simulink model "MRAC_P1_DZ"  (R2019b)
settings: Solver=VariableStepAuto  StartTime=0.0  StopTime=2000  RelTol=1e-3
undefined symbols (not defined in the file): sigbuilder_block
libraries: slctrlblks x3, simulink x2
settings Model: Creator=Henry  LastModifiedBy=Kevin
settings SFSimCC: CustomCodeUndefinedFunction=UseInterfaceOnly

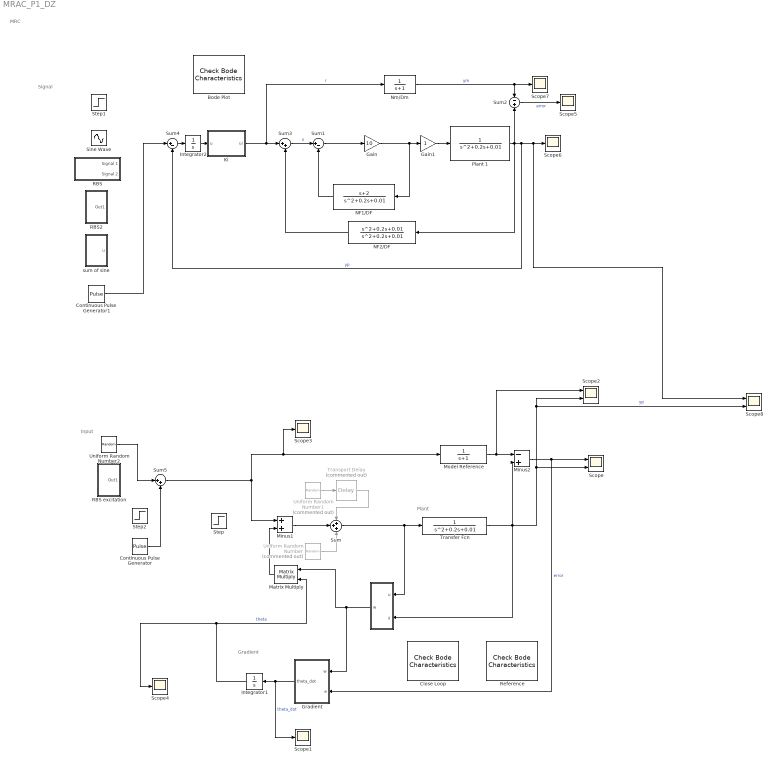
== system MRAC_P1_DZ ==
  note: Plant
  note: Gradient
  note: Signal
  note: MRC
  note: Input
  " " : Subsystem
  Bode Plot : slctrlblks/Model Verification/Check Bode  Characteristics  InstantiateOnLoad=on  SaveOperatingPoints=off  LinearizationIOs={'/Gain1', 1, 'in', 'off', '';'/Plant 1', 1, 'out', 'on', ''}  LinearizeAt=SnapshotTimes  SnapshotTimes=[0]  TriggerType=rising  SampleTime=auto  RateConversionMethod=zoh  PreWarpFreq=10  UseExactDelayModel=off  UseFullBlockNameLabels=off  UseBusSignalLabels=off  enabled=on  stopWhenAssertionFail=off  export=off  ViewDlgPos=[1981 -205.666666666667 1445.33333333333 714]  OpenViewOnLoad=off  LaunchViewOnOpen=off  FrequencyUnits=rad/s  MagnitudeUnits=dB  PhaseUnits=deg  TimeUnits=seconds  EnableUpperBound=off  UpperBoundFrequencies=[]  UpperBoundMagnitudes=[]  EnableLowerBound=off  LowerBoundFrequencies=[]  LowerBoundMagnitudes=[]
      settings: SourceProductName=Simulink Control Design
  Close Loop : slctrlblks/Model Verification/Check Bode  Characteristics  InstantiateOnLoad=on  SaveOperatingPoints=off  LinearizationIOs={'/Transfer Fcn', 1, 'out', 'off', '';'/Minus1', 1, 'in', 'off', ''}  LinearizeAt=SnapshotTimes  SnapshotTimes=[0]  TriggerType=rising  SampleTime=auto  RateConversionMethod=zoh  PreWarpFreq=10  UseExactDelayModel=off  UseFullBlockNameLabels=off  UseBusSignalLabels=off  enabled=on  stopWhenAssertionFail=off  export=off  ViewDlgPos=[100 200 510 390]  OpenViewOnLoad=off  LaunchViewOnOpen=on  FrequencyUnits=rad/s  MagnitudeUnits=dB  PhaseUnits=deg  TimeUnits=seconds  EnableUpperBound=off  UpperBoundFrequencies=[]  UpperBoundMagnitudes=[]  EnableLowerBound=off  LowerBoundFrequencies=[]  LowerBoundMagnitudes=[]
      settings: SourceProductName=Simulink Control Design
  Continuous Pulse Generator : DiscretePulseGenerator  PulseType=Time based  Period=100  PulseWidth=50
  Continuous Pulse Generator1 : DiscretePulseGenerator  PulseType=Time based  Period=100  PulseWidth=50
  Gain : Gain  Gain=10
  Gain1 : Gain
  Gradient : MATLAB Function  TreatAsAtomicUnit=on
  Integrator1 : Integrator
  Integrator2 : Integrator
  Ki : MATLAB Function  TreatAsAtomicUnit=on
  Matrix Multiply : Product  Multiplication=Matrix(*)
  Minus1 : Sum
  Minus2 : Sum  Inputs=-+
  Model Reference : TransferFcn  Denominator=[1 1]
  NF1/DF : TransferFcn  Numerator=[1 2]  Denominator=[1 0.2 0.01]
  NF2/DF : TransferFcn  Numerator=[1 0.2 0.01]  Denominator=[1 0.2 0.01]
  "Nm/Dm " : TransferFcn  Denominator=[1 1]
  Plant 1 : TransferFcn  Denominator=[1 ,0.2 ,0.01]
  "RBS " : Subsystem  Tag=STV Subsys  LoadFcn=sigbuilder_block('load');  StartFcn=sigbuilder_block('start');  StopFcn=sigbuilder_block('stop');  ClipboardFcn=sigbuilder_block('clipboard');  mask(Sigbuilder block){tuvar=[0:10]}
      mask help: Simulink:masks:SigbuilderBlock_MD
      mask init:
      | if ~strcmp(get_param(bdroot(gcbh),'SimulationStatus'),'stopped') tuvar = sigbuilder_block('maskInit'); end
      settings: CopyFcn=sigbuilder_block('copy');  DeleteFcn=sigbuilder_block('delete');  ModelCloseFcn=sigbuilder_block('modelClose');  PreSaveFcn=sigbuilder_block('preSave');  PauseFcn=sigbuilder_block('pause');  ContinueFcn=sigbuilder_block('continue');  NameChangeFcn=sigbuilder_block('namechange');  OpenFcn=sigbuilder_block('open',[215 62.5 550.5 362.5 ]);  CloseFcn=sigbuilder_block('close');
      mask Display: plot(0, 0, 100, 100,[2, 2, 32, 32, 2], [68, 8, 8, 68, 68],[32, 2], [38, 38], [32, 19, 2],[53, 60, 44], [32, 17, 17, 2],[16, 16, 31, 31]);txt = getActiveGroup(gcbh);text(2, 100, txt,'verticalAlignment', 'top');
  RBS excitation : Subsystem
  RBS2 : Subsystem
  Reference : slctrlblks/Model Verification/Check Bode  Characteristics  InstantiateOnLoad=on  SaveOperatingPoints=off  LinearizationIOs={'/Model Reference', 1, 'out', 'off', '';'/Step', 1, 'in', 'off', ''}  LinearizeAt=SnapshotTimes  SnapshotTimes=[0]  TriggerType=rising  SampleTime=auto  RateConversionMethod=zoh  PreWarpFreq=10  UseExactDelayModel=off  UseFullBlockNameLabels=off  UseBusSignalLabels=off  enabled=on  stopWhenAssertionFail=off  export=off  ViewDlgPos=[100 200 510 390]  OpenViewOnLoad=off  LaunchViewOnOpen=on  FrequencyUnits=rad/s  MagnitudeUnits=dB  PhaseUnits=deg  TimeUnits=seconds  EnableUpperBound=off  UpperBoundFrequencies=[]  UpperBoundMagnitudes=[]  EnableLowerBound=off  LowerBoundFrequencies=[]  LowerBoundMagnitudes=[]
      settings: SourceProductName=Simulink Control Design
  Scope : Scope  NumInputPorts=2
  Scope{1,3..7} (6 alike) : Scope
  Scope2 : Scope  NumInputPorts=2
  Scope8 : Scope  NumInputPorts=2
  Sine Wave : Sin  Frequency=0.1  SampleTime=0
  Step : Step  SampleTime=0
  Step1 : Step  SampleTime=0
  Step2 : Step  SampleTime=0
  Sum : Sum  Inputs=+++
  Sum1 : Sum  Inputs=|+-
  Sum2 : Sum  Inputs=-+
  Sum3 : Sum  Inputs=|++
  Sum4 : Sum  Inputs=|+-
  Sum5 : Sum  Inputs=|++
  Transfer Fcn : TransferFcn  Denominator=[1 ,0.2 ,0.01]
  Transport Delay : TransportDelay  Commented=on  DelayTime=150
  Uniform Random Number : UniformRandomNumber  Commented=on  SampleTime=0.05
  Uniform Random Number1 : UniformRandomNumber  Commented=on  Minimum=-5  Maximum=5  SampleTime=0.05
  Uniform Random Number2 : UniformRandomNumber  Minimum=-0.08  Maximum=0.08  SampleTime=1
  sum of sine : Subsystem
  wires:
  Model Reference/1 -> Scope2/1, Minus2/1
  Transfer Fcn/1 -> " "/2("y "), Scope8/2, Scope2/2, Scope/2, Minus2/2  "yp"
  Sum5/1 -> Minus1/1, Scope3/1, Model Reference/1
  Sum/1 -> " "/1("u "), Transfer Fcn/1
  Matrix Multiply/1 -> Minus1/2
  Gradient/1(theta_dot) -> Scope1/1, Integrator1/1  "theta_dot"
  " "/1(w) -> Gradient/1(w), Matrix Multiply/1
  Minus2/1 -> Scope/1, Gradient/2(e)  "error"
  Integrator1/1 -> Matrix Multiply/2, Scope4/1  "theta"
  Uniform Random Number/1 -> Sum/3
  Minus1/1 -> Sum/2
  Uniform Random Number1/1 -> Transport Delay/1
  Transport Delay/1 -> Sum/1
  NF1/DF/1 -> Sum1/2
  NF2/DF/1 -> Sum3/2
  Sum1/1 -> Gain/1
  Gain/1 -> Gain1/1, NF1/DF/1
  Sum4/1 -> Integrator2/1
  "Nm/Dm "/1 -> Scope7/1, Sum2/1  "ym"
  Gain1/1 -> Plant 1/1
  Ki/1(ui) -> "Nm/Dm "/1, Sum3/1  "r"
  Continuous Pulse Generator1/1 -> Sum4/1
  Sum3/1 -> Sum1/1  "u"
  Integrator2/1 -> Ki/1(u)
  Plant 1/1 -> Scope8/1, Scope6/1, Sum4/2, NF2/DF/1, Sum2/2  "yp"
  Sum2/1 -> Scope5/1  "error"
  Continuous Pulse Generator/1 -> Sum5/2
  Uniform Random Number2/1 -> Sum5/1

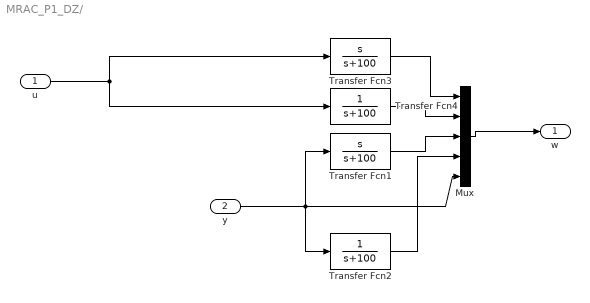
== system MRAC_P1_DZ/  ==
  "u " : Inport
  "y " : Inport  Port=2
  Mux : Mux  Inputs=5
  Transfer Fcn1 : TransferFcn  Numerator=[1 0]  Denominator=[1 100]
  Transfer Fcn2 : TransferFcn  Denominator=[1 100]
  Transfer Fcn3 : TransferFcn  Numerator=[1 0]  Denominator=[1 100]
  Transfer Fcn4 : TransferFcn  Denominator=[1 100]
  w : Outport
  wires:
  Transfer Fcn1/1 -> Mux/3
  "u "/1 -> Transfer Fcn3/1, Transfer Fcn4/1
  Mux/1 -> w/1
  "y "/1 -> Mux/5, Transfer Fcn2/1, Transfer Fcn1/1
  Transfer Fcn2/1 -> Mux/4
  Transfer Fcn3/1 -> Mux/1
  Transfer Fcn4/1 -> Mux/2

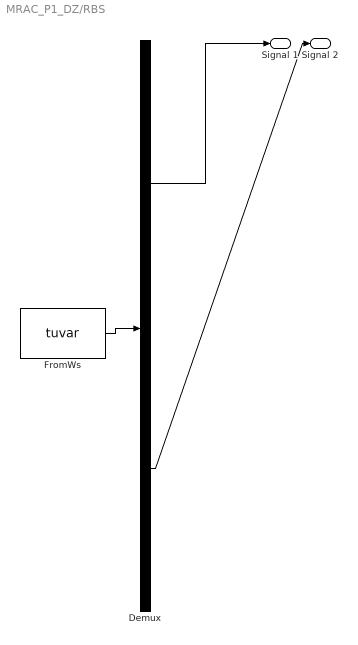
== system MRAC_P1_DZ/RBS  ==
  Demux : Demux  Tag=STV Demux  Outputs=2
  FromWs : FromWorkspace  Tag=STV FromWs  VariableName=tuvar  SampleTime=0
      SigBuilderData=|
      | common.afterFinalStr = 'Extrapolate'
      | common.sampleTime = 0
      | dataSet.timeRange = [0 10]
      | dataSet.name = 'Group 1'
      | sbobj.Groups.Name = 'Group 1'
      | sbobj.Groups.Signals(1).Name = 'Signal 1'
      | sbobj.Groups.Signals(1).XData = [0 4 4 6 6 10]
      | sbobj.Groups.Signals(1).YData = [0 0 1 1 0 0]
      | sbobj.Groups.Signals(2).Name = 'Signal 2'
      | sbobj.Groups.Signals(2).XData = [0 0.2 0.2 0.3 0.3 0.5 0.5 0.7 0.7 1 1 1.1 1.1 1.3 1.3 1.4 1.4 1.5 1.5 1.7 1.7 2.1 2.1 2.2 2.2 2.7 2.7 2.8 2.8 2.9 2.9 3 3 3.1 3.1 3.5 3.5 3.7 3.7 3.8 3.8 3.9 3.9 4.2 4.2 4.4 4.4 4.7 4.7 5 5 5.1 5.1 5.3 5.3 5.6 5.6 5.7 5.7 5.8 5.8 5.9 5.9 6 6 6.1 6.1 6.2 6.2 6.7 6.7 7 7 7.1 7.1 7.2 7.2 7.3 7.3 7.4 7.4 7.5 7.5 7.8 7.8 7.9 7.9 8.1 8.1 8.5 8.5 8.6 8.6 8.8 8.8 8.9 8.9 9 9 9.2 9.2 9.5 9.5 9.6 9.6 9.7 9.7 10]
      | sbobj.Groups.Signals(2).YData = [1 1 0 0 1 1 0 0 1 1 0 0 1 1 0 0 1 1 0 0 1 1 0 0 1 1 0 0 1 1 0 0 1 1 0 0 1 1 0 0 1 1 0 0 1 1 0 0 1 1 0 0 1 1 0 0 1 1 0 0 1 1 0 0 1 1 0 0 1 1 0 0 1 1 0 0 1 1 0 0 1 1 0 0 1 1 0 0 1 1 0 0 1 1 0 0 1 1 0 0 1 1 0 0 1 1 0 0]
  Signal 1 : Outport  Tag=STV Outport
  Signal 2 : Outport  Tag=STV Outport  Port=2
  wires:
  Demux/1 -> Signal 1/1
  FromWs/1 -> Demux/1
  Demux/2 -> Signal 2/1

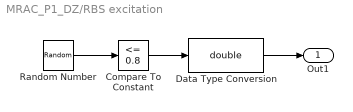
== system MRAC_P1_DZ/RBS excitation ==
  Compare To Constant : simulink/Logic and Bit Operations/Compare To Constant  relop=<=  const=0.8  OutDataTypeStr=boolean
  Data Type Conversion : DataTypeConversion  OutDataTypeStr=double
  Random Number : RandomNumber  Mean=1  SampleTime=10
  Out1 : Outport
  wires:
  Random Number/1 -> Compare To Constant/1
  Compare To Constant/1 -> Data Type Conversion/1
  Data Type Conversion/1 -> Out1/1

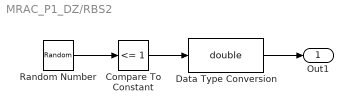
== system MRAC_P1_DZ/RBS2 ==
  Compare To Constant : simulink/Logic and Bit Operations/Compare To Constant  relop=<=  const=1  OutDataTypeStr=boolean
  Data Type Conversion : DataTypeConversion  OutDataTypeStr=double
  Random Number : RandomNumber  Mean=1  SampleTime=10
  Out1 : Outport
  wires:
  Random Number/1 -> Compare To Constant/1
  Compare To Constant/1 -> Data Type Conversion/1
  Data Type Conversion/1 -> Out1/1

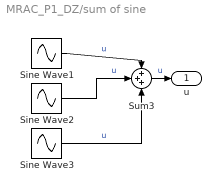
== system MRAC_P1_DZ/sum of sine ==
  Sine Wave1 : Sin  Frequency=0.1  Phase=0.1  SampleTime=0
  Sine Wave2 : Sin  SampleTime=0
  Sine Wave3 : Sin  Frequency=2  SampleTime=0
  Sum3 : Sum  Inputs=+++
  u : Outport
  wires:
  Sine Wave3/1 -> Sum3/3  "u"
  Sine Wave1/1 -> Sum3/1  "u"
  Sum3/1 -> u/1  "u"
  Sine Wave2/1 -> Sum3/2  "u"

== matlab function MRAC_P1_DZ/Gradient ==
  data: w input; theta_dot output; e input
function theta_dot = fcn(w, e)
alpha = 0.02;
I = eye(5);
gamma = alpha*I;

%deadzone implementation
delta= 0.1;
if abs(e) > delta
    theta_dot = -gamma*w*e;
else
    theta_dot = [0 0 0 0 0]';
end

== matlab function MRAC_P1_DZ/Ki ==
  data: u input; ui output
function ui = fcn(u)
 coder.extrinsic("ss","place","matsplit",'ctrb');
% [b2, b1, b0, a1, a0] = matsplit(theta);
ui = 0;
A = [0 1; -0.01 -0.2];
B = [0 1]';
C = [1 0];

o = [0 0]';
A1 = [A o;C 0];
B1 = [B;0];
p = [-.1+0.69805i -.1-0.69805i -1];
K1 = place(A1,B1,p);
Ki = [K1(3)];
ui = Ki*u;
